simulink model "ThreePhaseInvStarLoad"  (R2014a)
settings: Solver=ode23tb  StartTime=0.0  StopTime=2  RelTol=1e-3
libraries: powerlib x20
settings Model: Creator=ninad gaikawad  LastModifiedBy=ninad gaikawad

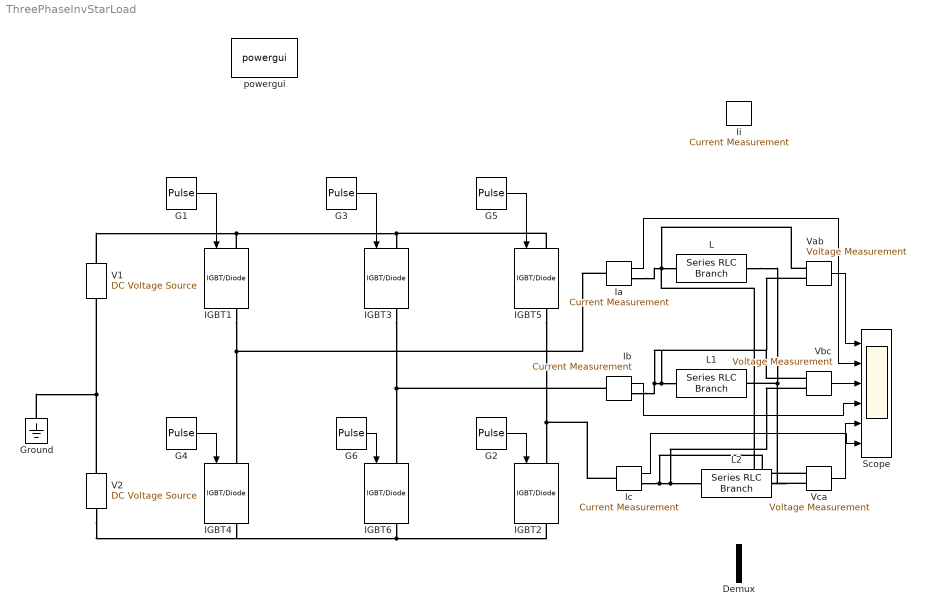
== system ThreePhaseInvStarLoad ==
  Demux : Demux  Outputs=2
  G1 : DiscretePulseGenerator  PulseType=Time based  Period=0.02  PulseWidth=50
  G2 : DiscretePulseGenerator  PulseType=Time based  Period=0.02  PulseWidth=50  PhaseDelay=2/150+0.01
  G3 : DiscretePulseGenerator  PulseType=Time based  Period=0.02  PulseWidth=50  PhaseDelay=1/150
  G4 : DiscretePulseGenerator  PulseType=Time based  Period=0.02  PulseWidth=50  PhaseDelay=0.01
  G5 : DiscretePulseGenerator  PulseType=Time based  Period=0.02  PulseWidth=50  PhaseDelay=2/150
  G6 : DiscretePulseGenerator  PulseType=Time based  Period=0.02  PulseWidth=50  PhaseDelay=1/150+0.01
  Ground : powerlib/Elements/Ground  LConnTagsString=a
  IGBT{1..6} (6 alike) : powerlib/Power Electronics/IGBT//Diode  Ron=1e-3  Rs=1e5  Cs=inf  Measurements=on
  Ia : powerlib/Measurements/Current Measurement  PhasorSimulation=off  OutputType=Complex  PSBequivalent=0
  Ib : powerlib/Measurements/Current Measurement  PhasorSimulation=off  OutputType=Complex  PSBequivalent=0
  Ic : powerlib/Measurements/Current Measurement  PhasorSimulation=off  OutputType=Complex  PSBequivalent=0
  Ii : powerlib/Measurements/Current Measurement  PhasorSimulation=off  OutputType=Complex  PSBequivalent=0
  L : powerlib/Elements/Series RLC Branch  LConnTagsString=__new0  RConnTagsString=__new0  BranchType=RL  Resistance=1  Inductance=0.01  SetiL0=off  InitialCurrent=0  Capacitance=1e-6  Setx0=off  InitialVoltage=0  Measurements=None
  L1 : powerlib/Elements/Series RLC Branch  LConnTagsString=__new0  RConnTagsString=__new0  BranchType=RL  Resistance=1  Inductance=0.01  SetiL0=off  InitialCurrent=0  Capacitance=1e-6  Setx0=off  InitialVoltage=0  Measurements=None
  L2 : powerlib/Elements/Series RLC Branch  LConnTagsString=__new0  RConnTagsString=__new0  BranchType=RL  Resistance=1  Inductance=0.01  SetiL0=off  InitialCurrent=0  Capacitance=1e-6  Setx0=off  InitialVoltage=0  Measurements=None
  Scope : Scope  NumInputPorts=6
      settings: YMin=-5~-5~-5~-5~-5~-5  YMax=5~5~5~5~5~5
  V1 : powerlib/Electrical Sources/DC Voltage Source  Amplitude=150  Measurements=None
  V2 : powerlib/Electrical Sources/DC Voltage Source  Amplitude=150  Measurements=None
  Vab : powerlib/Measurements/Voltage Measurement  PhasorSimulation=off  OutputType=Complex  PSBequivalent=0
  Vbc : powerlib/Measurements/Voltage Measurement  PhasorSimulation=off  OutputType=Complex  PSBequivalent=0
  Vca : powerlib/Measurements/Voltage Measurement  PhasorSimulation=off  OutputType=Complex  PSBequivalent=0
  powergui : powerlib/powergui  Priority=1  SimulationMode=Continuous  SolverType=Tustin  SampleTime=50e-6  frequency=60  SPID=off  DisableSnubberDevices=off  DisableRonSwitches=off  DisableVfSwitches=off  SwTol=0  Interpol=off  DisplayEquations=off  Ts=0  methode=off  frequencyindice=0  Pbase=100e6  ErrMax=1e-4  Iterations=50  UnitsV=kV  UnitsW=MW  FunctionMessages=off  echomessages=off  HookPort=off  EnableUseOfTLC=off  x0status=blocks  RestoreLinks=warning  ResistiveCurrentMeasurement=off  Frange=[0:2:500]  Ylog=off  Xlog=on  ShowGrid=off  save=off  variable=ZData  structure=0  ZoomFFT=off  StartTime=0.0  cycles=1  DisplayStyle=1  fundamental=60  FreqAxis=off  MaxFrequency=1000  frequencyindicesteady=1  RmsSteady=1  display=off
  wires:
  G1/1 -> IGBT1/1
  G3/1 -> IGBT3/1
  G5/1 -> IGBT5/1
  G2/1 -> IGBT2/1
  G6/1 -> IGBT6/1
  G4/1 -> IGBT4/1
  ? -> Demux/1
  Vab/1 -> Scope/1
  Vbc/1 -> Scope/3
  Vca/1 -> Scope/5
  Ia/1 -> Scope/2
  Ib/1 -> Scope/4
  Ic/1 -> Scope/6
  connections:
  IGBT1/RConn1 -- Ia/LConn1 -- IGBT4/LConn1
  IGBT5/RConn1 -- Ic/LConn1 -- IGBT2/LConn1
  IGBT1/LConn1 -- V1/RConn1 -- IGBT5/LConn1 -- IGBT3/LConn1
  IGBT6/RConn1 -- V2/LConn1 -- IGBT4/RConn1 -- IGBT2/RConn1
  V2/RConn1 -- V1/LConn1 -- Ground/LConn1
  IGBT3/RConn1 -- Ib/LConn1 -- IGBT6/LConn1
  L/LConn1 -- L2/LConn1 -- L1/LConn1
  Ic/RConn1 -- Vca/LConn1 -- Vbc/LConn2 -- L2/RConn1
  Ib/RConn1 -- Vab/LConn2 -- Vbc/LConn1 -- L1/RConn1
  Ia/RConn1 -- Vca/LConn2 -- Vab/LConn1 -- L/RConn1
